simulink model "Binarization"  (R2013b)
settings: Solver=ode45  StartTime=0.0  StopTime=1000  RelTol=1e-3
InitFcn:
  | %% DSPBuilder Start
  | alt_dspbuilder_update_model(bdroot)
  | %% DSPBuilder End
libraries: allblocks_alteradspbuilder2 x27
settings Model: Creator=Given_Jiang  LastModifiedBy=Given_Jiang

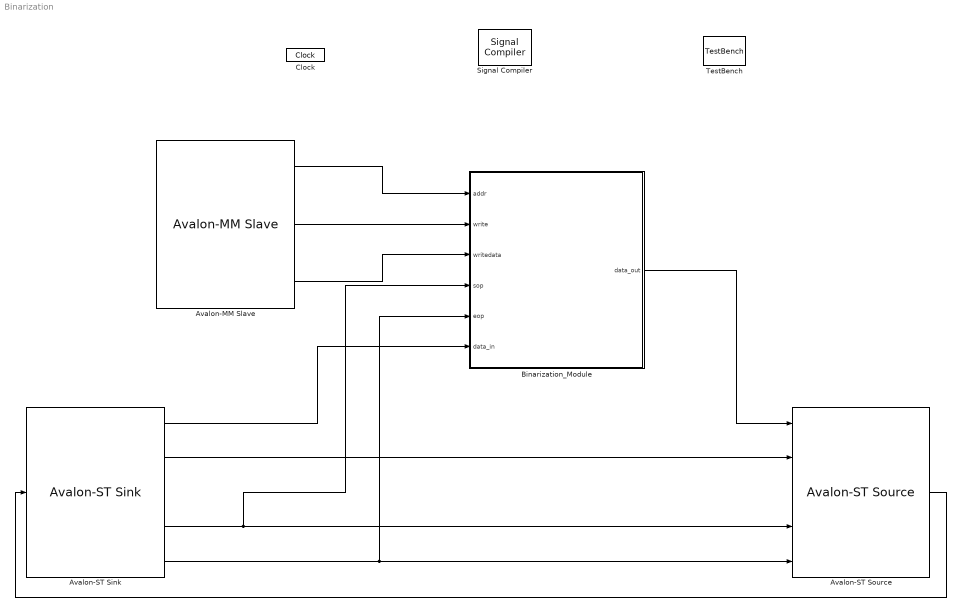
== system Binarization ==
  Avalon-MM Slave : allblocks_alteradspbuilder2/Avalon-MM Slave  iofile=E:\FPGA\SOC\Quartus\quartus\dsp_builder\design\VIP_LIB\Binarization\tb_Binarization\Binarization_Avalon-MM+Slave_address.salt,E:\FPGA\SOC\Quartus\quartus\dsp_builder\design\VIP_LIB\Binarization\tb_Binarization\Binarization_Avalon-MM+Slave_write.salt,E:\FPGA\SOC\Quartus\quartus\dsp_builder\design\VIP_LIB\Binarization\tb_Binarization\Binarization_Avalon-MM+Slave_writedata.salt,  SpecifyClock=off  addrWidth=2  addrAlignment=Dynamic  addrType=Write  BusType=Unsigned Integer  bwl=32  bwr=0  byteEnable=off  flowCtrl=off  pipeline=off  waitStateFormat=Fixed  readWaitStateCycles=0  writeWaitStateCycles=1  readLatencyFormat=Fixed  readLatencyCycles=0  burst=off  maxBurst=4  irq=off  receiveBeginTransfer=off  useChipSelect=off  externalType=Inferred  PORTTYPE=Output
  Avalon-ST Sink : allblocks_alteradspbuilder2/Avalon-ST Sink  iofile=E:\FPGA\SOC\Quartus\quartus\dsp_builder\design\VIP_LIB\Binarization\tb_Binarization\Binarization_Avalon-ST+Sink_data.salt,E:\FPGA\SOC\Quartus\quartus\dsp_builder\design\VIP_LIB\Binarization\tb_Binarization\Binarization_Avalon-ST+Sink_valid.salt,E:\FPGA\SOC\Quartus\quartus\dsp_builder\design\VIP_LIB\Binarization\tb_Binarization\Binarization_Avalon-ST+Sink_ready.capture,E:\FPGA\SOC\Quartus\quartus\dsp_builder\design\VIP_LIB\Binarization\tb_Binarization\Binarization_Avalon-ST+Sink_startofpacket.salt,E:\FPGA\SOC\Quartus\quartus\dsp_builder\design\VIP_LIB\Binarization\tb_Binarization\Binarization_Avalon-ST+Sink_endofpacket.salt,  SpecifyClock=off  BusType=Unsigned Integer  bwl=24  bwr=0  symbolWidth=8  symbolsPerBeat=3  numOfChannels=0  numOfErrorDescriptors=0  endOfPacket=on  startOfPacket=on  empty=off  readyLatency=1  externalType=Inferred  PORTTYPE=Output
  Avalon-ST Source : allblocks_alteradspbuilder2/Avalon-ST Source  iofile=E:\FPGA\SOC\Quartus\quartus\dsp_builder\design\VIP_LIB\Binarization\tb_Binarization\Binarization_Avalon-ST+Source_data.capture,E:\FPGA\SOC\Quartus\quartus\dsp_builder\design\VIP_LIB\Binarization\tb_Binarization\Binarization_Avalon-ST+Source_valid.capture,E:\FPGA\SOC\Quartus\quartus\dsp_builder\design\VIP_LIB\Binarization\tb_Binarization\Binarization_Avalon-ST+Source_ready.salt,E:\FPGA\SOC\Quartus\quartus\dsp_builder\design\VIP_LIB\Binarization\tb_Binarization\Binarization_Avalon-ST+Source_startofpacket.capture,E:\FPGA\SOC\Quartus\quartus\dsp_builder\design\VIP_LIB\Binarization\tb_Binarization\Binarization_Avalon-ST+Source_endofpacket.capture,  SpecifyClock=off  BusType=Unsigned Integer  bwl=24  bwr=0  symbolWidth=8  symbolsPerBeat=3  numOfChannels=0  numOfErrorDescriptors=0  endOfPacket=on  startOfPacket=on  empty=off  readyLatency=1  externalType=Inferred  PORTTYPE=Input
  Binarization_Module : Subsystem
  Clock : allblocks_alteradspbuilder2/Clock  ClockPeriod=7.5  ClockPeriodUnit=ns  SampleTime=1  ResetLatency=0  ResetRegisterCascadeDepth=0  SimulationStartCycle=5  PhaseOffset=0  Reset=aclr  ResetType=Active Low  Export=off
  Signal Compiler : allblocks_alteradspbuilder2/Signal Compiler  DeviceFamily=Cyclone V  DeviceName=AUTO  DisableEarlyHDLGeneration=off  EnableSignalTap=off  SignalTapDepth=128  UseBoardBlock=off  StpUseDefaultClock=on  StpClock=Clock  ExportDir=E:\FPGA\SOC\Quartus\quartus\dsp_builder
  TestBench : allblocks_alteradspbuilder2/TestBench  enable=on  advancedMode=on  modelSimGui=on  maxDisplayErrors=10  mismatchErrorLevel=Error  simdatafile=E:\FPGA\SOC\Quartus\quartus\dsp_builder\design\VIP_LIB\Binarization\tb_Binarization\Binarization.simdata.tcl
  wires:
  Avalon-ST Sink/2 -> Avalon-ST Source/2
  Avalon-ST Source/3 -> Avalon-ST Sink/3
  Avalon-ST Sink/4 -> Binarization_Module/4(sop), Avalon-ST Source/4
  Avalon-ST Sink/5 -> Binarization_Module/5(eop), Avalon-ST Source/5
  Avalon-ST Sink/1 -> Binarization_Module/6(data_in)
  Avalon-MM Slave/1 -> Binarization_Module/1(addr)
  Avalon-MM Slave/2 -> Binarization_Module/2(write)
  Avalon-MM Slave/3 -> Binarization_Module/3(writedata)
  Binarization_Module/1(data_out) -> Avalon-ST Source/1

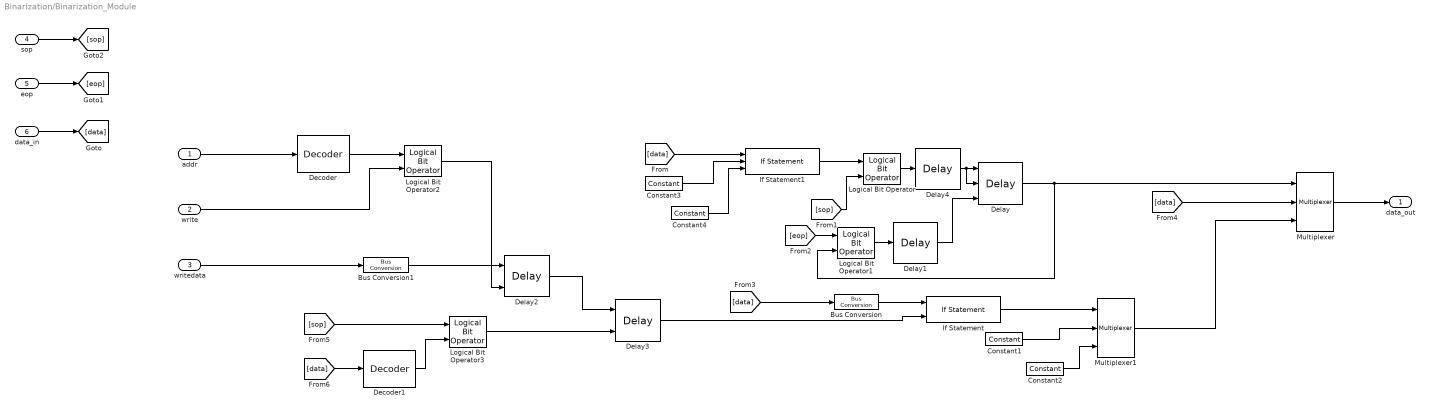
== system Binarization/Binarization_Module ==
  addr : Inport
  write : Inport  Port=2
  writedata : Inport  Port=3
  sop : Inport  Port=4
  eop : Inport  Port=5
  data_in : Inport  Port=6
  Bus Conversion : allblocks_alteradspbuilder2/Bus Conversion  BusType=Unsigned Integer  ibwl=24  ibwr=1  bwl=8  bwr=1  bitToConnectToOutputLSB=0  round=off  saturate=off  pipeline_display=0
  Bus Conversion1 : allblocks_alteradspbuilder2/Bus Conversion  BusType=Unsigned Integer  ibwl=24  ibwr=1  bwl=8  bwr=1  bitToConnectToOutputLSB=0  round=off  saturate=off  pipeline_display=0
  Constant1 : allblocks_alteradspbuilder2/Constant  mask_cst=0  BusType=Unsigned Integer  bwl=24  bwr=0  roundMode=Truncate  satMode=Wrap  SpecifyClock=off  allowFloatingPointOverride=on  logOutputs=off  logFile=E:\FPGA\SOC\Quartus\quartus\dsp_builder\design\VIP_LIB\Binarization\tb_Binarization\Binarization_Binarization%5FModule_Constant1.fixedpointlog
  Constant2 : allblocks_alteradspbuilder2/Constant  mask_cst=16777215  BusType=Unsigned Integer  bwl=24  bwr=0  roundMode=Truncate  satMode=Wrap  SpecifyClock=off  allowFloatingPointOverride=on  logOutputs=off  logFile=E:\FPGA\SOC\Quartus\quartus\dsp_builder\design\VIP_LIB\Binarization\tb_Binarization\Binarization_Binarization%5FModule_Constant2.fixedpointlog
  Constant3 : allblocks_alteradspbuilder2/Constant  mask_cst=0  BusType=Unsigned Integer  bwl=24  bwr=0  roundMode=Truncate  satMode=Wrap  SpecifyClock=off  allowFloatingPointOverride=on  logOutputs=off  logFile=E:\FPGA\SOC\Quartus\quartus\dsp_builder\design\VIP_LIB\Binarization\tb_Binarization\Binarization_Binarization%5FModule_Constant3.fixedpointlog
  Constant4 : allblocks_alteradspbuilder2/Constant  mask_cst=15  BusType=Unsigned Integer  bwl=24  bwr=0  roundMode=Truncate  satMode=Wrap  SpecifyClock=off  allowFloatingPointOverride=on  logOutputs=off  logFile=E:\FPGA\SOC\Quartus\quartus\dsp_builder\design\VIP_LIB\Binarization\tb_Binarization\Binarization_Binarization%5FModule_Constant4.fixedpointlog
  Decoder : allblocks_alteradspbuilder2/Decoder  BusType=Unsigned Integer  bwl=2  bwr=2  registered=on  pipeline_display=1  value=1
  Decoder1 : allblocks_alteradspbuilder2/Decoder  BusType=Unsigned Integer  bwl=24  bwr=2  registered=off  pipeline_display=0  value=15
  Delay : allblocks_alteradspbuilder2/Delay  pipeline=1  pipeline_display=1  ClockPhase=1  use_ena=on  use_sclr=on  allowFloatingPointOverride=on  logOutputs=off  logFile=E:\FPGA\SOC\Quartus\quartus\dsp_builder\design\VIP_LIB\Binarization\tb_Binarization\Binarization_Binarization%5FModule_Delay.fixedpointlog  use_init=on  reset_value=0
  Delay1 : allblocks_alteradspbuilder2/Delay  pipeline=1  pipeline_display=1  ClockPhase=1  use_ena=off  use_sclr=off  allowFloatingPointOverride=on  logOutputs=off  logFile=E:\FPGA\SOC\Quartus\quartus\dsp_builder\design\VIP_LIB\Binarization\tb_Binarization\Binarization_Binarization%5FModule_Delay1.fixedpointlog  use_init=off  reset_value=0
  Delay2 : allblocks_alteradspbuilder2/Delay  pipeline=1  pipeline_display=1  ClockPhase=1  use_ena=on  use_sclr=off  allowFloatingPointOverride=on  logOutputs=off  logFile=E:\FPGA\SOC\Quartus\quartus\dsp_builder\design\VIP_LIB\Binarization\tb_Binarization\Binarization_Binarization%5FModule_Delay2.fixedpointlog  use_init=on  reset_value=127
  Delay3 : allblocks_alteradspbuilder2/Delay  pipeline=1  pipeline_display=1  ClockPhase=1  use_ena=on  use_sclr=off  allowFloatingPointOverride=on  logOutputs=off  logFile=E:\FPGA\SOC\Quartus\quartus\dsp_builder\design\VIP_LIB\Binarization\tb_Binarization\Binarization_Binarization%5FModule_Delay3.fixedpointlog  use_init=on  reset_value=127
  Delay4 : allblocks_alteradspbuilder2/Delay  pipeline=1  pipeline_display=1  ClockPhase=1  use_ena=off  use_sclr=off  allowFloatingPointOverride=on  logOutputs=off  logFile=E:\FPGA\SOC\Quartus\quartus\dsp_builder\design\VIP_LIB\Binarization\tb_Binarization\Binarization_Binarization%5FModule_Delay4.fixedpointlog  use_init=off  reset_value=0
  If Statement : allblocks_alteradspbuilder2/If Statement  user_inputs=2  if_expression=a>b  BusType=Unsigned Integer  bwl=8  bwr=0  pipeline_display=1  use_else_output=off  use_elseif_input=off
  If Statement1 : allblocks_alteradspbuilder2/If Statement  user_inputs=3  if_expression=(a=b)&(a~c)  BusType=Unsigned Integer  bwl=24  bwr=0  pipeline_display=1  use_else_output=off  use_elseif_input=off
  Logical Bit Operator{,1..3} (4 alike) : allblocks_alteradspbuilder2/Logical Bit Operator  LogicalOperator=AND  user_inputs=2  pipeline_display=0
  Multiplexer : allblocks_alteradspbuilder2/Multiplexer  numInputs=2  pipeline=0  oneHot=off  pipeline_display=0  use_ena=off  use_aclr=off  allowFloatingPointOverride=on  logOutputs=off  logFile=E:\FPGA\SOC\Quartus\quartus\dsp_builder\design\VIP_LIB\Binarization\tb_Binarization\Binarization_Binarization%5FModule_Multiplexer.fixedpointlog
  Multiplexer1 : allblocks_alteradspbuilder2/Multiplexer  numInputs=2  pipeline=0  oneHot=off  pipeline_display=0  use_ena=off  use_aclr=off  allowFloatingPointOverride=on  logOutputs=off  logFile=E:\FPGA\SOC\Quartus\quartus\dsp_builder\design\VIP_LIB\Binarization\tb_Binarization\Binarization_Binarization%5FModule_Multiplexer1.fixedpointlog
  data_out : Outport
  wires:
  If Statement1/1 -> Logical Bit Operator/1
  Delay/1 -> Logical Bit Operator1/2, Multiplexer/1
  [data] -> If Statement1/1
  [sop] -> Logical Bit Operator/2
  [data] -> Bus Conversion/1
  Delay3/1 -> If Statement/2
  Bus Conversion/1 -> If Statement/1
  If Statement/1 -> Multiplexer1/1
  Constant1/1 -> Multiplexer1/2
  Multiplexer1/1 -> Multiplexer/3
  [data] -> Multiplexer/2
  Multiplexer/1 -> data_out/1
  Constant2/1 -> Multiplexer1/3
  Constant3/1 -> If Statement1/2
  Constant4/1 -> If Statement1/3
  [eop] -> Logical Bit Operator1/1
  Logical Bit Operator1/1 -> Delay1/1
  Delay1/1 -> Delay/3
  addr/1 -> Decoder/1
  Decoder/1 -> Logical Bit Operator2/1
  write/1 -> Logical Bit Operator2/2
  [data] -> Decoder1/1
  [sop] -> Logical Bit Operator3/1
  Decoder1/1 -> Logical Bit Operator3/2
  Logical Bit Operator2/1 -> Delay2/2
  Delay2/1 -> Delay3/1
  Logical Bit Operator3/1 -> Delay3/2
  writedata/1 -> Bus Conversion1/1
  Bus Conversion1/1 -> Delay2/1
  data_in/1 -> [data]
  eop/1 -> [eop]
  sop/1 -> [sop]
  Logical Bit Operator/1 -> Delay4/1
  Delay4/1 -> Delay/2, Delay/1
